simulink model "testemplanner_cs"  (R2020a)
settings: Solver=ode5  StartTime=0.0  StopTime=24  FixedStep=1/1000  RelTol=1e-3
PreLoadFcn:
  | mbxruntime.callbacks.PreLoadFcn(bdroot);
PostLoadFcn:
  | mbxruntime.callbacks.PostLoadFcn(bdroot);
InitFcn:
  | mbxruntime.callbacks.InitFcn(bdroot);
StartFcn:
  | mbxruntime.callbacks.StartFcn(bdroot);
StopFcn:
  | mbxruntime.callbacks.StopFcn(bdroot);
model workspace (MAT data in the model file):
  mbox_table : object (value not decoded)
  model_closed = 0
  sim_status = 0
values from neighbouring files (symbols this model uses):
  c_factor = 43.75    [emplanner_init.m]
  cf = -175016    [emplanner_init.m]
  cr = -130634    [emplanner_init.m]
  global_path_x = [0.057304 1.05668625507 2.05480936558 3.05165624935 4.04722112279 5.04150235808 6.03449985569 7.02621407764 8.01664569183 9.00579544113 9.99366409523 10.9802524329 ... (3001 elements, 3001x1)]    [global_path.mat]
  global_path_y = [8.29 8.29 8.29 8.29 8.29 8.29 8.29 8.29 8.29 8.29 8.29 8.29 ... (3001 elements, 3001x1)]    [global_path.mat]
  KD_PID_distance = 0.0    (= 0)    [emplanner_init.m]
  KD_PID_speed = 0    [emplanner_init.m]
  KI_PID_distance = 0.0    (= 0)    [emplanner_init.m]
  KI_PID_speed = 0    [emplanner_init.m]
  KP_PID_distance = 0.5    [emplanner_init.m]
  KP_PID_speed = 1.8    [emplanner_init.m]
  la = 1.265    [emplanner_init.m]
  lb = 2.947-1.265    (= 1.682)    [emplanner_init.m]
  LQR_K1 = k(:,1)'    [emplanner_init.m]
  LQR_K2 = k(:,2)'    [emplanner_init.m]
  LQR_K3 = k(:,3)'    [emplanner_init.m]
  LQR_K4 = k(:,4)'    [emplanner_init.m]
  m = 2020    [emplanner_init.m]
  rack_displacement = [-39.14 , -37.2 , -35.29 , -33.43 , -31.6 , -29.81 , -28.06 , -26.34 , -24.66 ,      -23.01 , -21.38 , -19.79 , -18.23 , -16.69 , -15.18 , -13.7 , -12.23 , -10.8 , -9.38 , -7.98 ,     -6.61 , -5.25 , -3.91 , -2.59 , -1.29 , 0 , 1.27 , 2.54 , 3.78 , 5.02 , 6.24 , 7.46 , 8.66 ,      9.86 , 11.05 , 12.24 , 13.41 , 14.59 , 15.76 , 16.92 , 18.09 , 19.25 , 20.42 , 21.59 , 22.76 ,      23.93 , 25.11 , 26 ...(+26 chars)    [emplanner_init.m]
  right_wheel_ground = [-70 ,-67.2 , -64.4 , -61.6 , -58.8 , -56 , -53.2 , -50.4 , -47.6 , -44.8 , -42 ,      -39.2 , -36.4 , -33.6 , -30.8 , -28 , -25.2 , -22.4 , -19.6 , -16.8 , -14 , -11.2 , -8.4 , -5.6 ,      -2.8 , 0 , 2.8 , 5.6 , 8.4 , 11.2 , 14 , 16.8 , 19.6 , 22.4 , 25.2 , 28 , 30.8 , 33.6 , 36.4 ,      39.2 , 42 , 44.8 , 47.6 , 50.4 , 53.2 , 56 , 58.8 , 61.6 , 64.4 , 67.2 , 70 ]    [emplanner_init.m]
  vx_break_point = zeros(1,5000)    [emplanner_init.m]
undefined symbols (not defined in the file or in its folder): aubr, DiscIntNeverNeededParam, tablebr, vubr
libraries: PreScanSimulinkLibrary x9, Solver_SF x1, simulink_extras x1
(part 2 of 9)

== system testemplanner_cs/Audi_A8_Sedan_1/control module2 ==
  location_info : Inport
  planning_result : Inport  Port=2
  control_predict_time[s] : Inport  Port=3
  current_time[s] : Inport  Port=4
  Trigger : TriggerPort  TriggerType=function-call  VariantControl=Variant  PortDimensions=1
  Bus Selector1 : BusSelector  OutputSignals=host_x,host_y,host_heading_xy,host_vx,host_vy,host_yawrate,host_speed
  Bus Selector2 : BusSelector  OutputSignals=trajectory_x_gcs,trajectory_y_gcs,trajectory_heading_gcs,trajectory_kappa_gcs,trajectory_speed_gcs,trajectory_accel_gcs,trajectory_time_gcs
  MATLAB Function1 : MATLAB Function  TreatAsAtomicUnit=on
  MATLAB Function2 : MATLAB Function  Commented=on  TreatAsAtomicUnit=on
  control main : Subsystem
  lateral_steer_sw : Outport
  throttle : Outport  Port=2
  brake : Outport  Port=3
  debug_control : Outport  Port=4
  wires:
  [accel] -> control main/13(accelerate_desire[m/s^2])
  [x_r] -> control main/8(xr_desire[m])
  [theta_r] -> control main/10(thetar_desire[rad])
  [y_r] -> control main/9(yr_desire[m])
  [speed] -> control main/12(speed_desire[m/s])
  [kappa_r] -> control main/11(kappar_desire[m^-1])
  MATLAB Function1/4(kappar) -> [kappa_r]
  MATLAB Function1/3(thetar) -> [theta_r]
  MATLAB Function1/2(yr) -> [y_r]
  MATLAB Function1/5(vr) -> [speed]
  MATLAB Function1/6(ar) -> [accel]
  MATLAB Function1/1(xr) -> [x_r]
  current_time[s]/1 -> MATLAB Function1/8(current_time)
  Bus Selector2/1 -> MATLAB Function1/1(trajectory_x)  "<trajectory_x_gcs>"
  Bus Selector2/2 -> MATLAB Function1/2(trajectory_y)  "<trajectory_y_gcs>"
  Bus Selector2/3 -> MATLAB Function1/3(trajectory_heading)  "<trajectory_heading_gcs>"
  Bus Selector2/4 -> MATLAB Function1/4(trajectory_kappa)  "<trajectory_kappa_gcs>"
  Bus Selector2/5 -> MATLAB Function1/5(trajectory_speed)  "<trajectory_speed_gcs>"
  Bus Selector2/6 -> MATLAB Function1/6(trajectory_accel)  "<trajectory_accel_gcs>"
  Bus Selector2/7 -> MATLAB Function1/7(trajectory_time)  "<trajectory_time_gcs>"
  control main/3(brake) -> brake/1
  control main/1(lateral_steer_sw) -> lateral_steer_sw/1
  control main/4(debug_control) -> debug_control/1
  planning_result/1 -> Bus Selector2/1
  control_predict_time[s]/1 -> control main/14(control_predict_time[s])
  location_info/1 -> Bus Selector1/1
  Bus Selector1/3 -> control main/3(host_heading_xy[rad])  "<host_heading_xy>"
  Bus Selector1/6 -> control main/6(host_yawrate[rad/s])  "<host_yawrate>"
  Bus Selector1/1 -> control main/1(host_x[m])  "<host_x>"
  control main/2(throttle) -> throttle/1
  Bus Selector1/7 -> control main/7(host_speed[m/s])  "<host_speed>"
  Bus Selector1/2 -> control main/2(host_y[m])  "<host_y>"
  Bus Selector1/4 -> control main/4(host_vx[m/s])  "<host_vx>"
  Bus Selector1/5 -> control main/5(host_vy[m/s])  "<host_vy>"

== system testemplanner_cs/Audi_A8_Sedan_1/control module3 ==
  location_info : Inport
  planning_result : Inport  Port=2
  control_predict_time[s] : Inport  Port=3
  current_time : Inport  Port=4
  Trigger : TriggerPort  TriggerType=function-call  VariantControl=Variant  PortDimensions=1
  Bus Selector : BusSelector  OutputSignals=trajectory_x_final[m],trajectory_y_final[m],trajectory_heading_final[rad],trajectory_kappa_final[1/m],trajectory_velocity_final[m/s],trajectory_accelerate_final[m/s^2],trajectory_time_final[m/s^2]
  Bus Selector1 : BusSelector  OutputSignals=host_x,host_y,host_heading_xy,host_vx,host_vy,host_yawrate,host_speed
  MATLAB Function : MATLAB Function  TreatAsAtomicUnit=on
  control main : Subsystem
  lateral_steer_sw : Outport
  throttle : Outport  Port=2
  brake : Outport  Port=3
  debug_control : Outport  Port=4
  wires:
  [trajecotory_x] -> MATLAB Function/1(trajectory_x)
  [trajecotory_y] -> MATLAB Function/2(trajectory_y)
  [trajecotory_heading] -> MATLAB Function/3(trajectory_heading)
  [trajecotory_kappa] -> MATLAB Function/4(trajectory_kappa)
  [trajecotory_speed] -> MATLAB Function/5(trajectory_speed)
  [trajecotory_accel] -> MATLAB Function/6(trajectory_accel)
  [trajecotory_time] -> MATLAB Function/7(trajectory_time)
  Bus Selector/7 -> [trajecotory_time]  "<trajectory_time_final[m/s^2]>"
  Bus Selector/6 -> [trajecotory_accel]  "<trajectory_accelerate_final[m/s^2]>"
  Bus Selector/5 -> [trajecotory_speed]  "<trajectory_velocity_final[m/s]>"
  Bus Selector/4 -> [trajecotory_kappa]  "<trajectory_kappa_final[1/m]>"
  Bus Selector/3 -> [trajecotory_heading]  "<trajectory_heading_final[rad]>"
  Bus Selector/2 -> [trajecotory_y]  "<trajectory_y_final[m]>"
  Bus Selector/1 -> [trajecotory_x]  "<trajectory_x_final[m]>"
  planning_result/1 -> Bus Selector/1
  current_time/1 -> MATLAB Function/8(current_time)
  MATLAB Function/1(xr) -> control main/8(xr_desire[m])
  MATLAB Function/2(yr) -> control main/9(yr_desire[m])
  MATLAB Function/3(thetar) -> control main/10(thetar_desire[rad])
  MATLAB Function/4(kappar) -> control main/11(kappar_desire[m^-1])
  MATLAB Function/5(vr) -> control main/12(speed_desire[m/s])
  MATLAB Function/6(ar) -> control main/13(accelerate_desire[m/s^2])
  control main/3(brake) -> brake/1
  control main/1(lateral_steer_sw) -> lateral_steer_sw/1
  control main/4(debug_control) -> debug_control/1
  control_predict_time[s]/1 -> control main/14(control_predict_time[s])
  location_info/1 -> Bus Selector1/1
  Bus Selector1/3 -> control main/3(host_heading_xy[rad])  "<host_heading_xy>"
  Bus Selector1/6 -> control main/6(host_yawrate[rad/s])  "<host_yawrate>"
  Bus Selector1/1 -> control main/1(host_x[m])  "<host_x>"
  control main/2(throttle) -> throttle/1
  Bus Selector1/7 -> control main/7(host_speed[m/s])  "<host_speed>"
  Bus Selector1/2 -> control main/2(host_y[m])  "<host_y>"
  Bus Selector1/4 -> control main/4(host_vx[m/s])  "<host_vx>"
  Bus Selector1/5 -> control main/5(host_vy[m/s])  "<host_vy>"

== system testemplanner_cs/Audi_A8_Sedan_1/decision&planning module ==
  note: 灰色的函数为通用算法函数，可以在多个模块复用
  location_info : Inport
  routine_info : Inport  Port=2
  perceptiong_result : Inport  Port=3
  current_time : Inport  Port=4
  pre_planning_result : Inport  Port=5
  Trigger : TriggerPort  TriggerType=function-call  VariantControl=Variant  PortDimensions=1
  Bus Creator : BusCreator  Inputs=1
  Bus Creator1 : BusCreator  Inputs=4
  EM Planner : Subsystem
  EM_planner1 : Subsystem  Commented=on
  referenceline provider : Subsystem
  planning_result : Outport
  debug_planning : Outport  Port=2
  wires:
  [planning_info] -> planning_result/1
  referenceline provider/2(referenceline_y[m]) -> [referenceline_y]
  routine_info/1 -> [routine_info]
  [routine_info] -> referenceline provider/2(routine_info)
  referenceline provider/5(referenceline_debug) -> [referenceline_debug]
  referenceline provider/4(referenceline_kappa[rad/m]) -> [referenceline_kappa]
  referenceline provider/1(referenceline_x[m]) -> [referenceline_x]
  [Location_info] -> referenceline provider/1(location_info)
  location_info/1 -> [Location_info]
  referenceline provider/3(referenceline_heading[rad]) -> [referenceline_heading]
  [referenceline_debug] -> Bus Creator/1  "debug_referenceline"
  Bus Creator/1 -> debug_planning/1
  perceptiong_result/1 -> [perceptiong_result]
  [referenceline_kappa] -> Bus Creator1/4
  [referenceline_x] -> Bus Creator1/1
  [referenceline_heading] -> Bus Creator1/3
  [referenceline_y] -> Bus Creator1/2
  Bus Creator1/1 -> [referenceline_info]
  [Location_info] -> EM Planner/2(location info)
  [referenceline_info] -> EM Planner/1(referenceline info)
  [perceptiong_result] -> EM Planner/3(perception info)
  current_time/1 -> [current_time]
  pre_planning_result/1 -> [pre_planning_result]
  [current_time] -> EM Planner/5(current time)
  [pre_planning_result] -> EM Planner/4(pre_planning info)
  EM Planner/1(EM Planner result) -> [planning_info]

== system testemplanner_cs/Audi_A8_Sedan_1/location module ==
  host_x[m] : Inport
  host_y[m] : Inport  Port=2
  host_heading_xy[rad] : Inport  Port=3
  host_vx[m/s] : Inport  Port=4
  host_vy[m/s] : Inport  Port=5
  host_yawrate[rad/s] : Inport  Port=6
  host_speed[m/s] : Inport  Port=7
  host_ax[m·s(-2)] : Inport  Port=8
  host_ay[m·s(-2)] : Inport  Port=9
  Bus Creator : BusCreator  Inputs=9
  location_Info : Outport
  wires:
  host_yawrate[rad/s]/1 -> Bus Creator/6  "host_yawrate"
  host_vy[m/s]/1 -> Bus Creator/5  "host_vy"
  host_heading_xy[rad]/1 -> Bus Creator/3  "host_heading_xy"
  host_speed[m/s]/1 -> Bus Creator/7  "host_speed"
  Bus Creator/1 -> location_Info/1
  host_y[m]/1 -> Bus Creator/2  "host_y"
  host_x[m]/1 -> Bus Creator/1  "host_x"
  host_vx[m/s]/1 -> Bus Creator/4  "host_vx"
  host_ay[m·s(-2)]/1 -> Bus Creator/9  "host_ay"
  host_ax[m·s(-2)]/1 -> Bus Creator/8  "host_ax"

== system testemplanner_cs/Audi_A8_Sedan_1/routine module ==
  Bus Creator : BusCreator  Inputs=2
  Constant : Constant  Value=global_path_x
  Constant1 : Constant  Value=global_path_y
  global_path_info : Outport
  wires:
  Constant/1 -> [global_path_x]
  Constant1/1 -> [global_path_y]
  [global_path_x] -> Bus Creator/1  "global_path_x"
  [global_path_y] -> Bus Creator/2  "global_path_y"
  Bus Creator/1 -> global_path_info/1

== system testemplanner_cs/Box_1/Dynamics_Empty ==
  note: For state mode 'Dynamic' positions
      | are not taken into account, as they
      | are computed by integrating velocity.
      | Click annotation for Help.
  Ground_{1..9} (9 alike) : Ground
  MuxState : Subsystem  Tag=mux/State  mask(Empty Dynamics State Block){positioningmode=on, TimeStep=50/1000}
      mask prompts: positioningmode "Positioning Mode"; TimeStep "Auto Assigned: Time Step [s]"
      mask help:
      | Build the state of an actor based on user input.
      | The user can either use positioning mode or dynamics mode.
      | - When using positioning mode the position and orientation of the actor are set directly based on the input. Expected input is relative to the initial position and orientation of the actor. It's also possible to specify the velocity of the actor, though this input isn't used, only passed on.
      | - When using dynamics mode the position input is ignored. Expected input is velocity and orientation. The velocity is relative the current orientation of the actor, while orientation is relative to its initial orientation. The position of the actor is calculated based on the velocity and orientation given.
      settings: DeleteFcn=PreScanBlockDeleteFcn;
  State : Outport  Tag=outport/StateOutport  SampleTime=50/1000
  wires:
  MuxState/1(state) -> State/1
  Ground_1/1 -> MuxState/1(x [m])
  Ground_2/1 -> MuxState/2(y [m])
  Ground_3/1 -> MuxState/3(z [m])
  Ground_4/1 -> MuxState/4(dx [m/s])
  Ground_5/1 -> MuxState/5(dy [m/s])
  Ground_6/1 -> MuxState/6(dz [m/s])
  Ground_7/1 -> MuxState/7(R [rad])
  Ground_8/1 -> MuxState/8(P [rad])
  Ground_9/1 -> MuxState/9(Y [rad])

== system testemplanner_cs/Box_1/SELF_Demux ==
  SELF : Inport  OutDataTypeStr=Bus: PRESCAN_SELFSENSORDATA
  Bus Selector : BusSelector  OutputSignals=PositionX,PositionY,PositionZ,OrientationRoll,OrientationPitch,OrientationYaw,Velocity,Yaw_rate,Lat,Long,Alt
  Demux2 : Demux  Outputs=3
  Gain : Gain  Gain=180/pi
  Gain1 : Gain  Gain=180/pi
  Vector Concatenate1 : Concatenate  NumInputs=3
  compas converter : Subsystem
  x [m] : Outport
  y [m] : Outport  Port=2
  z [m] : Outport  Port=3
  rotx [deg] : Outport  Port=4
  roty [deg] : Outport  Port=5
  rotz [deg] : Outport  Port=6
  GPS lat [deg] : Outport  Port=7
  GPS long [deg] : Outport  Port=8
  GPS alt [m] : Outport  Port=9
  velocity [m/s] : Outport  Port=10
  heading [deg] : Outport  Port=11
  yaw rate [deg/s] : Outport  Port=12
  wires:
  Bus Selector/11 -> GPS alt [m]/1  "<Alt>"
  Bus Selector/10 -> GPS long [deg]/1  "<Long>"
  Bus Selector/9 -> GPS lat [deg]/1  "<Lat>"
  Bus Selector/8 -> Gain1/1  "<Yaw_rate>"
  Bus Selector/7 -> velocity [m/s]/1  "<Velocity>"
  Bus Selector/6 -> compas converter/1(rotz [rad]), Vector Concatenate1/3  "<OrientationYaw>"
  Bus Selector/5 -> Vector Concatenate1/2  "<OrientationPitch>"
  Bus Selector/4 -> Vector Concatenate1/1  "<OrientationRoll>"
  Vector Concatenate1/1 -> Gain/1
  Bus Selector/3 -> z [m]/1  "<PositionZ>"
  Bus Selector/2 -> y [m]/1  "<PositionY>"
  Bus Selector/1 -> x [m]/1  "<PositionX>"
  SELF/1 -> Bus Selector/1
  Gain/1 -> Demux2/1
  Demux2/1 -> rotx [deg]/1
  Demux2/2 -> roty [deg]/1
  Demux2/3 -> rotz [deg]/1
  compas converter/1(heading [deg]) -> heading [deg]/1
  Gain1/1 -> yaw rate [deg/s]/1

== system testemplanner_cs/Box_1/STATE_Box_1 ==
  State : Inport  SampleTime=TimeStep
  Bus Creator : BusCreator  Inputs=15  OutDataTypeStr=Bus: PRESCAN_STATEACTUATORDATA  NonVirtualBus=on
  Demux : Demux  Outputs=15
  iniBODYAngles wrtVEH [rad] : Constant  Value=[Roll0 Pitch0 0]  SampleTime=TimeStep
  iniVEHAngles wrtGLOB [rad] : Constant  Value=[0 0 Yaw0]  SampleTime=TimeStep
  iniVEHposition wrtGLOB [m] : Constant  Value=[x0 y0 z0]  SampleTime=TimeStep
  state2FullState : PreScanSimulinkLibrary/state2FullState  SystemSampleTime=-1  Latency=0  AutoFrameSizeCalculation=off
  StateBus : Outport  OutDataTypeStr=Bus: PRESCAN_STATEACTUATORDATA
  wires:
  Bus Creator/1 -> StateBus/1
  State/1 -> state2FullState/1
  state2FullState/1 -> Demux/1
  iniVEHposition wrtGLOB [m]/1 -> state2FullState/2
  iniBODYAngles wrtVEH [rad]/1 -> state2FullState/3
  iniVEHAngles wrtGLOB [rad]/1 -> state2FullState/4
  Demux/1 -> Bus Creator/1  "PositionX"
  Demux/2 -> Bus Creator/2  "PositionY"
  Demux/3 -> Bus Creator/3  "PositionZ"
  Demux/4 -> Bus Creator/4  "VelocityX"
  Demux/5 -> Bus Creator/5  "VelocityY"
  Demux/6 -> Bus Creator/6  "VelocityZ"
  Demux/7 -> Bus Creator/7  "AccelerationX"
  Demux/8 -> Bus Creator/8  "AccelerationY"
  Demux/9 -> Bus Creator/9  "AccelerationZ"
  Demux/10 -> Bus Creator/10  "OrientationRoll"
  Demux/11 -> Bus Creator/11  "OrientationPitch"
  Demux/12 -> Bus Creator/12  "OrientationYaw"
  Demux/13 -> Bus Creator/13  "AngularVelocityRoll"
  Demux/14 -> Bus Creator/14  "AngularVelocityPitch"
  Demux/15 -> Bus Creator/15  "AngularVelocityYaw"

== system testemplanner_cs/Audi_A8_Sedan_1/AIR_1_Demux/Activate_Switch ==
  BeamID : Inport
  Heading : Inport  Port=2
  Constant : Constant  Value=0
  Product1 : Product  RndMeth=Zero
  Relational Operator : RelationalOperator  Operator=~=  OutDataTypeStr=boolean  RndMeth=Nearest
  On/Off : Outport
  wires:
  Constant/1 -> Relational Operator/1
  Relational Operator/1 -> Product1/1
  BeamID/1 -> Relational Operator/2
  Product1/1 -> On/Off/1
  Heading/1 -> Product1/2

== system testemplanner_cs/Audi_A8_Sedan_1/AIR_1_Demux/Signal2ArrayOfSignals1 ==
  note: Set mask parameter VECTORLENGTH
      |  to MAXMESSAGES
  note: Initial state of Previous vector block
      | set to zeros(VECTORLENGTH,1)
  LoopIndex : Inport
  Element : Inport  Port=2
  Assignment : Assignment  IndexOptions=Index vector (port)  Indices=1  OutputSizes=1
  Previous vector : Memory  InitialCondition=zeros(VECTORLENGTH,1)  InheritSampleTime=on
  ArrayofElements : Outport
  wires:
  Element/1 -> Assignment/2
  LoopIndex/1 -> Assignment/3
  Previous vector/1 -> Assignment/1
  Assignment/1 -> ArrayofElements/1, Previous vector/1

== system testemplanner_cs/Audi_A8_Sedan_1/AIR_1_Demux/Signal2ArrayOfSignals2 ==
  note: Set mask parameter VECTORLENGTH
      |  to MAXMESSAGES
  note: Initial state of Previous vector block
      | set to zeros(VECTORLENGTH,1)
  LoopIndex : Inport
  Element : Inport  Port=2
  Assignment : Assignment  IndexOptions=Index vector (port)  Indices=1  OutputSizes=1
  Previous vector : Memory  InitialCondition=zeros(VECTORLENGTH,1)  InheritSampleTime=on
  ArrayofElements : Outport
  wires:
  Element/1 -> Assignment/2
  LoopIndex/1 -> Assignment/3
  Previous vector/1 -> Assignment/1
  Assignment/1 -> ArrayofElements/1, Previous vector/1

== system testemplanner_cs/Audi_A8_Sedan_1/AIR_1_Demux/Signal2ArrayOfSignals3 ==
  note: Set mask parameter VECTORLENGTH
      |  to MAXMESSAGES
  note: Initial state of Previous vector block
      | set to zeros(VECTORLENGTH,1)
  LoopIndex : Inport
  Element : Inport  Port=2
  Assignment : Assignment  IndexOptions=Index vector (port)  Indices=1  OutputSizes=1
  Previous vector : Memory  InitialCondition=zeros(VECTORLENGTH,1)  InheritSampleTime=on
  ArrayofElements : Outport
  wires:
  Element/1 -> Assignment/2
  LoopIndex/1 -> Assignment/3
  Previous vector/1 -> Assignment/1
  Assignment/1 -> ArrayofElements/1, Previous vector/1

== system testemplanner_cs/Audi_A8_Sedan_1/AIR_1_Demux/Signal2ArrayOfSignals4 ==
  note: Set mask parameter VECTORLENGTH
      |  to MAXMESSAGES
  note: Initial state of Previous vector block
      | set to zeros(VECTORLENGTH,1)
  LoopIndex : Inport
  Element : Inport  Port=2
  Assignment : Assignment  IndexOptions=Index vector (port)  Indices=1  OutputSizes=1
  Previous vector : Memory  InitialCondition=zeros(VECTORLENGTH,1)  InheritSampleTime=on
  ArrayofElements : Outport
  wires:
  Element/1 -> Assignment/2
  LoopIndex/1 -> Assignment/3
  Previous vector/1 -> Assignment/1
  Assignment/1 -> ArrayofElements/1, Previous vector/1

== system testemplanner_cs/Audi_A8_Sedan_1/AIR_1_Demux/Signal2ArrayOfSignals5 ==
  note: Set mask parameter VECTORLENGTH
      |  to MAXMESSAGES
  note: Initial state of Previous vector block
      | set to zeros(VECTORLENGTH,1)
  LoopIndex : Inport
  Element : Inport  Port=2
  Assignment : Assignment  IndexOptions=Index vector (port)  Indices=1  OutputSizes=1
  Previous vector : Memory  InitialCondition=zeros(VECTORLENGTH,1)  InheritSampleTime=on
  ArrayofElements : Outport
  wires:
  Element/1 -> Assignment/2
  LoopIndex/1 -> Assignment/3
  Previous vector/1 -> Assignment/1
  Assignment/1 -> ArrayofElements/1, Previous vector/1

== system testemplanner_cs/Audi_A8_Sedan_1/AIR_1_Demux/Signal2ArrayOfSignals6 ==
  note: Set mask parameter VECTORLENGTH
      |  to MAXMESSAGES
  note: Initial state of Previous vector block
      | set to zeros(VECTORLENGTH,1)
  LoopIndex : Inport
  Element : Inport  Port=2
  Assignment : Assignment  IndexOptions=Index vector (port)  Indices=1  OutputSizes=1
  Previous vector : Memory  InitialCondition=zeros(VECTORLENGTH,1)  InheritSampleTime=on
  ArrayofElements : Outport
  wires:
  Element/1 -> Assignment/2
  LoopIndex/1 -> Assignment/3
  Previous vector/1 -> Assignment/1
  Assignment/1 -> ArrayofElements/1, Previous vector/1

== system testemplanner_cs/Audi_A8_Sedan_1/Dynamics_UserSpecified/CarSim2PreScanSTATE ==
  CarSim_In : Inport
  D2R : Gain  Gain=pi/180
  Demux : Demux  Outputs=[3 3 3 -1]
  Demux1 : Demux  Outputs=3
  Demux2 : Demux  Outputs=3
  Demux3 : Demux  Outputs=3
  Demux4 : Demux  Outputs=28
  Gain : Gain  Gain=9.8
  Gain1 : Gain  Gain=9.8
  Terminator_{1..26} (26 alike) : Terminator
  Transformation_SprungMassCarSim2PreScan : Subsystem
  km|h_to_m|s : Gain  Gain=1/3.6
  x [m] : Outport
  y [m] : Outport  Port=2
  z [m] : Outport  Port=3
  dx [m/s] : Outport  Port=4
  dy [m/s] : Outport  Port=5
  dz [m/s] : Outport  Port=6
  R [rad] : Outport  Port=7
  P [rad] : Outport  Port=8
  Y [rad] : Outport  Port=9
  ax [m/s^2] : Outport  Port=10
  ay [m/s^2] : Outport  Port=11
  wires:
  Demux/4 -> Demux4/1
  Demux3/3 -> Y [rad]/1
  Demux3/2 -> P [rad]/1
  Demux3/1 -> R [rad]/1
  Demux2/3 -> dz [m/s]/1
  Demux2/2 -> dy [m/s]/1
  Demux2/1 -> dx [m/s]/1
  Demux1/3 -> z [m]/1
  Demux1/2 -> y [m]/1
  Demux1/1 -> x [m]/1
  Transformation_SprungMassCarSim2PreScan/1(Out1) -> Demux1/1
  Demux/1 -> Transformation_SprungMassCarSim2PreScan/1(In1)
  CarSim_In/1 -> Demux/1
  km|h_to_m|s/1 -> Demux2/1
  Demux/2 -> km|h_to_m|s/1
  Demux/3 -> D2R/1
  D2R/1 -> Demux3/1
  Demux4/28 -> Gain1/1
  Demux4/27 -> Gain/1
  Gain/1 -> ax [m/s^2]/1
  Gain1/1 -> ay [m/s^2]/1
  Demux4/1 -> Terminator_1/1
  Demux4/2 -> Terminator_2/1
  Demux4/3 -> Terminator_3/1
  Demux4/4 -> Terminator_4/1
  Demux4/5 -> Terminator_5/1
  Demux4/6 -> Terminator_6/1
  Demux4/7 -> Terminator_7/1
  Demux4/8 -> Terminator_8/1
  Demux4/9 -> Terminator_9/1
  Demux4/10 -> Terminator_10/1
  Demux4/11 -> Terminator_11/1
  Demux4/12 -> Terminator_12/1
  Demux4/13 -> Terminator_13/1
  Demux4/14 -> Terminator_14/1
  Demux4/15 -> Terminator_15/1
  Demux4/16 -> Terminator_16/1
  Demux4/17 -> Terminator_17/1
  Demux4/18 -> Terminator_18/1
  Demux4/19 -> Terminator_19/1
  Demux4/20 -> Terminator_20/1
  Demux4/21 -> Terminator_21/1
  Demux4/22 -> Terminator_22/1
  Demux4/23 -> Terminator_23/1
  Demux4/24 -> Terminator_24/1
  Demux4/25 -> Terminator_25/1
  Demux4/26 -> Terminator_26/1

== system testemplanner_cs/Audi_A8_Sedan_1/Dynamics_UserSpecified/MuxState ==
  note: mode: Dynamics
  note: mode: Positioning
  note: mode: Dynamics
      | VelVEHICLE
      | wrt VEH
  note: AnglesVEHICLE
      | wrtGLOB
  note: For state mode 'Dynamic' positions
      | are not taken into account, as they
      | are computed by integrating velocity.
      | Click annotation for Help.
  x [m] : Inport  SampleTime=TimeStep
  y [m] : Inport  Port=2  SampleTime=TimeStep
  z [m] : Inport  Port=3  SampleTime=TimeStep
  dx [m/s] : Inport  Port=4  SampleTime=TimeStep
  dy [m/s] : Inport  Port=5  SampleTime=TimeStep
  dz [m/s] : Inport  Port=6  SampleTime=TimeStep
  R [rad] : Inport  Port=7  SampleTime=TimeStep
  P [rad] : Inport  Port=8  SampleTime=TimeStep
  Y [rad] : Inport  Port=9  SampleTime=TimeStep
  Constant : Constant  DisableCoverage=on  Value=positioningmode
  Discrete-Time Integrator : DiscreteIntegrator  SampleTime=TimeStep  ICPrevOutput=DiscIntNeverNeededParam  ICPrevScaledInput=DiscIntNeverNeededParam
  Ground : Ground
  Ground1 : Ground
  Mux1 : Mux  Inputs=[3 3]
  Mux2 : Mux  Inputs=3
  Mux3 : Mux  Inputs=3
  Mux4 : Mux  Inputs=3
  Mux5 : Mux  Inputs=[3 3]
  Mux6 : Mux  Inputs=[6 3]
  Switch : Switch  Threshold=0.5
  Transformation_BODY2GLOBAL : PreScanSimulinkLibrary/Simple_Vehicle_Dynamics/Chassis/MuxDynState/Transformation_BODY2GLOBAL  SystemSampleTime=-1  Latency=0  AutoFrameSizeCalculation=off
  mux3 : Mux  Inputs=3
  state : Outport
  wires:
  Constant/1 -> Switch/2
  Mux6/1 -> state/1
  Mux4/1 -> Mux1/1
  Mux5/1 -> Switch/3
  Mux1/1 -> Switch/1
  Switch/1 -> Mux6/1  "PosVeh wrt  GLOB"
  P [rad]/1 -> Mux3/2
  R [rad]/1 -> Mux3/1
  dz [m/s]/1 -> Mux2/3
  dy [m/s]/1 -> Mux2/2
  dx [m/s]/1 -> Mux2/1
  z [m]/1 -> Mux4/3
  y [m]/1 -> Mux4/2
  x [m]/1 -> Mux4/1
  Ground1/1 -> mux3/2  "pitch"
  Y [rad]/1 -> mux3/3, Mux3/3  "yaw"
  Mux3/1 -> Mux6/2
  Transformation_BODY2GLOBAL/1 -> Discrete-Time Integrator/1, Mux5/2  "VelVEH wrt  GLOB"
  mux3/1 -> Transformation_BODY2GLOBAL/2
  Ground/1 -> mux3/1  "roll"
  Mux2/1 -> Mux1/2, Transformation_BODY2GLOBAL/1
  Discrete-Time Integrator/1 -> Mux5/1  "PosVEH wrt  GLOB"

== system testemplanner_cs/Audi_A8_Sedan_1/SELF_Demux/compas converter ==
  rotz [rad] : Inport
  cart2compas : Subsystem
  rad2deg : Gain  Gain=180/pi
  heading [deg] : Outport
  wires:
  rad2deg/1 -> cart2compas/1(Angle [deg])
  rotz [rad]/1 -> rad2deg/1
  cart2compas/1(heading [deg]) -> heading [deg]/1

== system testemplanner_cs/Audi_A8_Sedan_1/Trajectories/Traj2State1 ==
  Traj Org : Inport
  Offset : Inport  Port=2
  Add2 : Sum
  ApplyRotation : PreScanSimulinkLibrary/ApplyRotation  SystemSampleTime=-1  Latency=0  AutoFrameSizeCalculation=off
  ApplyRotation1 : PreScanSimulinkLibrary/ApplyRotation  SystemSampleTime=-1  Latency=0  AutoFrameSizeCalculation=off
  ApplyRotation2 : PreScanSimulinkLibrary/ApplyRotation  SystemSampleTime=-1  Latency=0  AutoFrameSizeCalculation=off
  Constant : Constant  Value=zeros(12,1)
  Mux : Mux  Inputs=6
  Mux1 : Mux  Inputs=2
  Mux{2,4..9} (7 alike) : Mux  Inputs=3
  Mux3 : Mux  Inputs=2
  Selector : Selector  InputPortWidth=6  IndexOptions=Index vector (dialog)  Indices=[4 5 6]  OutputSizes=1
  Selector1 : Selector  InputPortWidth=21  IndexOptions=Index vector (dialog)  Indices=[5]  OutputSizes=1
  Selector10 : Selector  InputPortWidth=21  IndexOptions=Index vector (dialog)  Indices=[2]  OutputSizes=1
  Selector11 : Selector  InputPortWidth=21  IndexOptions=Index vector (dialog)  Indices=[3]  OutputSizes=1
  Selector12 : Selector  InputPortWidth=21  IndexOptions=Index vector (dialog)  Indices=[1]  OutputSizes=1
  Selector13 : Selector  InputPortWidth=21  IndexOptions=Index vector (dialog)  Indices=[8]  OutputSizes=1
  Selector14 : Selector  InputPortWidth=21  IndexOptions=Index vector (dialog)  Indices=[9]  OutputSizes=1
  Selector15 : Selector  InputPortWidth=21  IndexOptions=Index vector (dialog)  Indices=[7]  OutputSizes=1
  Selector16 : Selector  InputPortWidth=21  IndexOptions=Index vector (dialog)  Indices=[14]  OutputSizes=1
  Selector17 : Selector  InputPortWidth=21  IndexOptions=Index vector (dialog)  Indices=[15]  OutputSizes=1
  Selector18 : Selector  InputPortWidth=21  IndexOptions=Index vector (dialog)  Indices=[13]  OutputSizes=1
  Selector19 : Selector  InputPortWidth=21  IndexOptions=Index vector (dialog)  Indices=[20]  OutputSizes=1
  Selector2 : Selector  InputPortWidth=21  IndexOptions=Index vector (dialog)  Indices=[6]  OutputSizes=1
  Selector20 : Selector  InputPortWidth=21  IndexOptions=Index vector (dialog)  Indices=[21]  OutputSizes=1
  Selector21 : Selector  InputPortWidth=21  IndexOptions=Index vector (dialog)  Indices=[19]  OutputSizes=1
  Selector3 : Selector  InputPortWidth=21  IndexOptions=Index vector (dialog)  Indices=[12]  OutputSizes=1
  Selector4 : Selector  InputPortWidth=21  IndexOptions=Index vector (dialog)  Indices=[17]  OutputSizes=1
  Selector5 : Selector  InputPortWidth=21  IndexOptions=Index vector (dialog)  Indices=[18]  OutputSizes=1
  Selector6 : Selector  InputPortWidth=21  IndexOptions=Index vector (dialog)  Indices=[16]  OutputSizes=1
  Selector7 : Selector  InputPortWidth=21  IndexOptions=Index vector (dialog)  Indices=[11]  OutputSizes=1
  Selector8 : Selector  InputPortWidth=21  IndexOptions=Index vector (dialog)  Indices=[10]  OutputSizes=1
  Selector9 : Selector  InputPortWidth=21  IndexOptions=Index vector (dialog)  Indices=[4]  OutputSizes=1
  Traj2State2 : Subsystem
  state : Outport
  wires:
  Mux9/1 -> ApplyRotation2/2, ApplyRotation1/2, ApplyRotation/2
  Selector20/1 -> Mux9/3
  Selector19/1 -> Mux9/2
  Selector21/1 -> Mux9/1
  Selector5/1 -> Mux8/3
  Selector4/1 -> Mux8/2
  Selector6/1 -> Mux8/1
  Mux8/1 -> Mux/6
  Mux6/1 -> ApplyRotation2/1
  Mux7/1 -> Mux/4
  ApplyRotation2/1 -> Mux/5
  Selector3/1 -> Mux7/3
  Selector7/1 -> Mux7/2
  Selector8/1 -> Mux7/1
  Mux4/1 -> Mux/2
  Mux5/1 -> ApplyRotation1/1
  ApplyRotation1/1 -> Mux/3
  Mux2/1 -> ApplyRotation/1
  ApplyRotation/1 -> Mux/1
  Selector2/1 -> Mux4/3
  Selector1/1 -> Mux4/2
  Selector9/1 -> Mux4/1
  Selector17/1 -> Mux6/3
  Selector16/1 -> Mux6/2
  Selector18/1 -> Mux6/1
  Selector14/1 -> Mux5/3
  Selector13/1 -> Mux5/2
  Selector15/1 -> Mux5/1
  Selector11/1 -> Mux2/3
  Selector10/1 -> Mux2/2
  Selector12/1 -> Mux2/1
  Mux3/1 -> Selector8/1, Selector7/1, Selector3/1, Selector18/1, Selector16/1, Selector17/1, Selector6/1, Selector20/1, Selector19/1, Selector21/1, Selector5/1, Selector4/1, Selector14/1, Selector13/1, Selector15/1, Selector2/1, Selector1/1, Selector9/1, Selector12/1, Selector10/1, Selector11/1
  Mux1/1 -> Add2/2
  Constant/1 -> Mux1/2
  Add2/1 -> Traj2State2/1(traj)
  Selector/1 -> Mux3/2
  Traj Org/1 -> Mux3/1
  Offset/1 -> Mux1/1, Selector/1
  Mux/1 -> Add2/1
  Traj2State2/1(state) -> state/1

== system testemplanner_cs/Audi_A8_Sedan_1/Trajectories/TrajCoGOffset ==
  State In : Inport
  Add : Sum  Inputs=+-+
  Add1 : Sum
  ApplyRotation : PreScanSimulinkLibrary/ApplyRotation  SystemSampleTime=-1  Latency=0  AutoFrameSizeCalculation=off
  ApplyRotation1 : PreScanSimulinkLibrary/ApplyRotation  SystemSampleTime=-1  Latency=0  AutoFrameSizeCalculation=off
  CoG Offset : Constant  Value=[0 0 CoGOffsetZ]
  Degrees to Radians : simulink_extras/Transformations/Degrees to Radians
  Demux1 : Demux  Outputs=[3 3 3]
  Mux : Mux  Inputs=[3 3 3]
  Orientation : Constant  Value=[InitRoll InitPitch 0]
  State Out : Outport
  wires:
  State In/1 -> Demux1/1
  Demux1/1 -> Add/1
  Add/1 -> Mux/1
  Demux1/3 -> Mux/3, Add1/2
  Mux/1 -> State Out/1
  Demux1/2 -> Mux/2
  Orientation/1 -> Degrees to Radians/1
  ApplyRotation/1 -> Add/3
  ApplyRotation1/1 -> Add/2
  Add1/1 -> ApplyRotation/2
  CoG Offset/1 -> ApplyRotation1/1, ApplyRotation/1
  Degrees to Radians/1 -> Add1/1, ApplyRotation1/2

== system testemplanner_cs/Audi_A8_Sedan_1/Trajectories/Trajectory_1 ==
  From Workspace : FromWorkspace  VariableName=trajectory  SampleTime=TimeStep  ZeroCross=off  OutputAfterFinalValue=Holding final value
  From Workspace1 : FromWorkspace  VariableName=trajectory  SampleTime=TimeStep  ZeroCross=off  OutputAfterFinalValue=Setting to zero
  Mux : Mux  Inputs=2
  Selector1 : Selector  InputPortWidth=24  IndexOptions=Index vector (dialog)  Indices=[7:18]  OutputSizes=1
  Selector9 : Selector  InputPortWidth=24  IndexOptions=Index vector (dialog)  Indices=[1:6]  OutputSizes=1
  trajectory : Outport
  wires:
  From Workspace/1 -> Selector9/1
  From Workspace1/1 -> Selector1/1
  Mux/1 -> trajectory/1
  Selector9/1 -> Mux/1
  Selector1/1 -> Mux/2

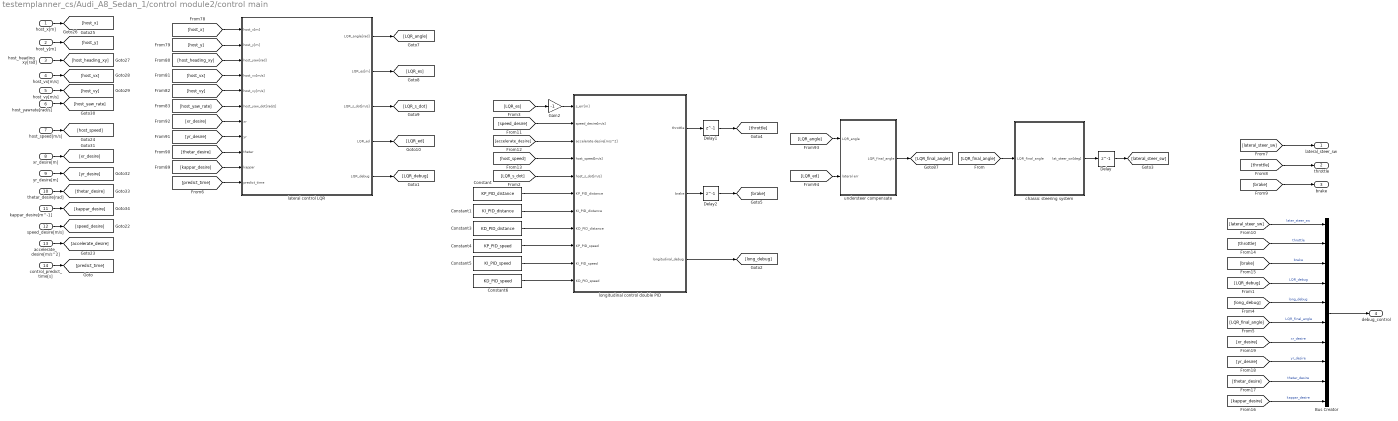
== system testemplanner_cs/Audi_A8_Sedan_1/control module2/control main ==
  host_x[m] : Inport
  host_y[m] : Inport  Port=2
  host_heading_xy[rad] : Inport  Port=3
  host_vx[m/s] : Inport  Port=4
  host_vy[m/s] : Inport  Port=5
  host_yawrate[rad/s] : Inport  Port=6
  host_speed[m/s] : Inport  Port=7
  xr_desire[m] : Inport  Port=8
  yr_desire[m] : Inport  Port=9
  thetar_desire[rad] : Inport  Port=10
  kappar_desire[m^-1] : Inport  Port=11
  speed_desire[m/s] : Inport  Port=12
  accelerate_desire[m/s^2] : Inport  Port=13
  control_predict_time[s] : Inport  Port=14
  Bus Creator : BusCreator  Inputs=10
  Constant : Constant  Value=KP_PID_distance
  Constant1 : Constant  Value=KI_PID_distance
  Constant3 : Constant  Value=KD_PID_distance
  Constant4 : Constant  Value=KP_PID_speed
  Constant5 : Constant  Value=KI_PID_speed
  Constant6 : Constant  Value=KD_PID_speed
  Delay : Delay  DelayLength=1
  Delay1 : Delay  DelayLength=1
  Delay2 : Delay  DelayLength=1
  Gain2 : Gain  Gain=-1
  chassic steering system : Subsystem
  lateral control LQR : Subsystem
  longitudinal control double PID : Subsystem
  understeer compensate : Subsystem
  lateral_steer_sw : Outport
  throttle : Outport  Port=2
  brake : Outport  Port=3
  debug_control : Outport  Port=4
  wires:
  [kappar_desire] -> Bus Creator/10  "kappar_desire"
  [thetar_desire] -> Bus Creator/9  "thetar_desire"
  [yr_desire] -> Bus Creator/8  "yr_desire"
  [xr_desire] -> Bus Creator/7  "xr_desire"
  Bus Creator/1 -> debug_control/1
  [LQR_final_angle] -> Bus Creator/6  "LQR_final_angle"
  [long_debug] -> Bus Creator/5  "long_debug"
  [LQR_debug] -> Bus Creator/4  "LQR_debug"
  [brake] -> Bus Creator/3  "brake"
  [throttle] -> Bus Creator/2  "throttle"
  [lateral_steer_sw] -> Bus Creator/1  "later_steer_sw"
  [brake] -> brake/1
  [throttle] -> throttle/1
  [lateral_steer_sw] -> lateral_steer_sw/1
  Delay2/1 -> [brake]
  Delay1/1 -> [throttle]
  Delay/1 -> [lateral_steer_sw]
  longitudinal control double PID/3(longitudinal_debug) -> [long_debug]
  lateral control LQR/5(LQR_debug) -> [LQR_debug]
  longitudinal control double PID/2(brake) -> Delay2/1
  longitudinal control double PID/1(throttle) -> Delay1/1
  chassic steering system/1(lat_steer_sw[deg]) -> Delay/1
  [LQR_final_angle] -> chassic steering system/1(LQR_final_angle)
  [LQR_es] -> Gain2/1
  Gain2/1 -> longitudinal control double PID/1(s_err[m])
  Constant6/1 -> longitudinal control double PID/11(KD_PID_speed)
  speed_desire[m/s]/1 -> [speed_desire]
  control_predict_time[s]/1 -> [predict_time]
  host_speed[m/s]/1 -> [host_speed]
  host_vy[m/s]/1 -> [host_vy]
  host_y[m]/1 -> [host_y]
  [host_yaw_rate] -> lateral control LQR/6(host_yaw_dot[rad/s])
  yr_desire[m]/1 -> [yr_desire]
  kappar_desire[m^-1]/1 -> [kappar_desire]
  host_yawrate[rad/s]/1 -> [host_yaw_rate]
  [kappar_desire] -> lateral control LQR/10(kappar)
  [host_heading_xy] -> lateral control LQR/3(host_yaw[rad])
  [thetar_desire] -> lateral control LQR/9(thetar)
  lateral control LQR/4(LQR_ed) -> [LQR_ed]
  [speed_desire] -> longitudinal control double PID/2(speed_desire[m/s])
  host_vx[m/s]/1 -> [host_vx]
  [predict_time] -> lateral control LQR/11(predict_time)
  [host_speed] -> longitudinal control double PID/4(host_speed[m/s])
  Constant4/1 -> longitudinal control double PID/9(KP_PID_speed)
  Constant5/1 -> longitudinal control double PID/10(KI_PID_speed)
  Constant3/1 -> longitudinal control double PID/8(KD_PID_distance)
  Constant/1 -> longitudinal control double PID/6(KP_PID_distance)
  lateral control LQR/3(LQR_s_dot[m/s]) -> [LQR_s_dot]
  [LQR_ed] -> understeer compensate/2(lateral err)
  host_heading_xy[rad]/1 -> [host_heading_xy]
  lateral control LQR/2(LQR_es[m]) -> [LQR_es]
  [host_vy] -> lateral control LQR/5(host_vy[m/s])
  xr_desire[m]/1 -> [xr_desire]
  [LQR_angle] -> understeer compensate/1(LQR_angle)
  [yr_desire] -> lateral control LQR/8(yr)
  [LQR_s_dot] -> longitudinal control double PID/5(host_s_dot[m/s])
  [host_y] -> lateral control LQR/2(host_y[m])
  accelerate_desire[m/s^2]/1 -> [accelerate_desire]
  [xr_desire] -> lateral control LQR/7(xr)
  [host_x] -> lateral control LQR/1(host_x[m])
  [accelerate_desire] -> longitudinal control double PID/3(accelerate desire[m/s^2])
  Constant1/1 -> longitudinal control double PID/7(KI_PID_distance)
  thetar_desire[rad]/1 -> [thetar_desire]
  [host_vx] -> lateral control LQR/4(host_vx[m/s])
  lateral control LQR/1(LQR_angle[rad]) -> [LQR_angle]
  understeer compensate/1(LQR_final_angle) -> [LQR_final_angle]
  host_x[m]/1 -> [host_x]

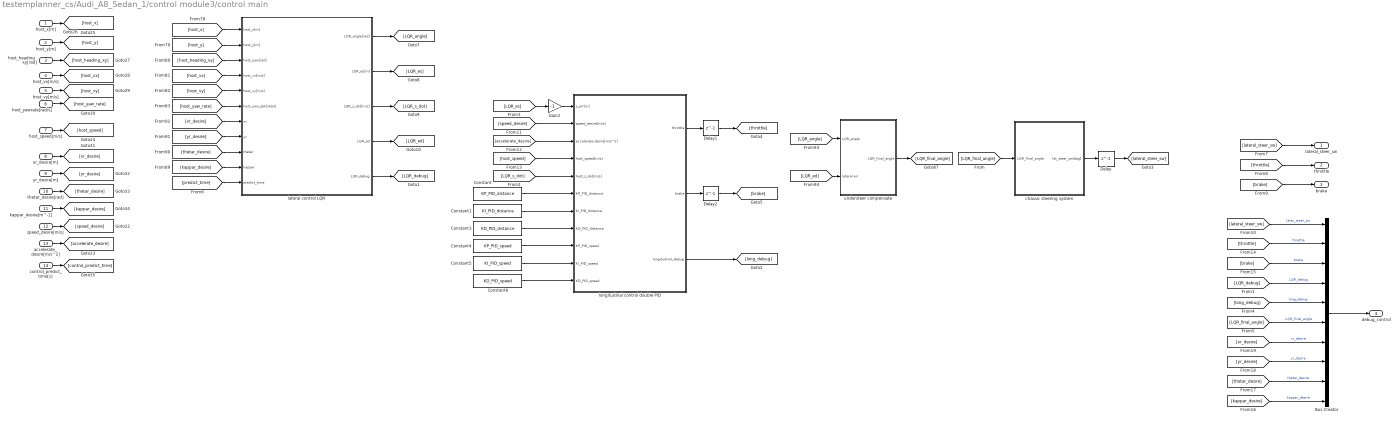
== system testemplanner_cs/Audi_A8_Sedan_1/control module3/control main ==
  host_x[m] : Inport
  host_y[m] : Inport  Port=2
  host_heading_xy[rad] : Inport  Port=3
  host_vx[m/s] : Inport  Port=4
  host_vy[m/s] : Inport  Port=5
  host_yawrate[rad/s] : Inport  Port=6
  host_speed[m/s] : Inport  Port=7
  xr_desire[m] : Inport  Port=8
  yr_desire[m] : Inport  Port=9
  thetar_desire[rad] : Inport  Port=10
  kappar_desire[m^-1] : Inport  Port=11
  speed_desire[m/s] : Inport  Port=12
  accelerate_desire[m/s^2] : Inport  Port=13
  control_predict_time[s] : Inport  Port=14
  Bus Creator : BusCreator  Inputs=10
  Constant : Constant  Value=KP_PID_distance
  Constant1 : Constant  Value=KI_PID_distance
  Constant3 : Constant  Value=KD_PID_distance
  Constant4 : Constant  Value=KP_PID_speed
  Constant5 : Constant  Value=KI_PID_speed
  Constant6 : Constant  Value=KD_PID_speed
  Delay : Delay  DelayLength=1
  Delay1 : Delay  DelayLength=1
  Delay2 : Delay  DelayLength=1
  Gain2 : Gain  Gain=-1
  chassic steering system : Subsystem
  lateral control LQR : Subsystem
  longitudinal control double PID : Subsystem
  understeer compensate : Subsystem
  lateral_steer_sw : Outport
  throttle : Outport  Port=2
  brake : Outport  Port=3
  debug_control : Outport  Port=4
  wires:
  [kappar_desire] -> Bus Creator/10  "kappar_desire"
  [thetar_desire] -> Bus Creator/9  "thetar_desire"
  [yr_desire] -> Bus Creator/8  "yr_desire"
  [xr_desire] -> Bus Creator/7  "xr_desire"
  Bus Creator/1 -> debug_control/1
  [LQR_final_angle] -> Bus Creator/6  "LQR_final_angle"
  [long_debug] -> Bus Creator/5  "long_debug"
  [LQR_debug] -> Bus Creator/4  "LQR_debug"
  [brake] -> Bus Creator/3  "brake"
  [throttle] -> Bus Creator/2  "throttle"
  [lateral_steer_sw] -> Bus Creator/1  "later_steer_sw"
  [brake] -> brake/1
  [throttle] -> throttle/1
  [lateral_steer_sw] -> lateral_steer_sw/1
  Delay2/1 -> [brake]
  Delay1/1 -> [throttle]
  Delay/1 -> [lateral_steer_sw]
  longitudinal control double PID/3(longitudinal_debug) -> [long_debug]
  lateral control LQR/5(LQR_debug) -> [LQR_debug]
  longitudinal control double PID/2(brake) -> Delay2/1
  longitudinal control double PID/1(throttle) -> Delay1/1
  chassic steering system/1(lat_steer_sw[deg]) -> Delay/1
  [LQR_final_angle] -> chassic steering system/1(LQR_final_angle)
  [LQR_es] -> Gain2/1
  Gain2/1 -> longitudinal control double PID/1(s_err[m])
  Constant6/1 -> longitudinal control double PID/11(KD_PID_speed)
  speed_desire[m/s]/1 -> [speed_desire]
  control_predict_time[s]/1 -> [control_predict_time]
  host_speed[m/s]/1 -> [host_speed]
  host_vy[m/s]/1 -> [host_vy]
  host_y[m]/1 -> [host_y]
  [host_yaw_rate] -> lateral control LQR/6(host_yaw_dot[rad/s])
  yr_desire[m]/1 -> [yr_desire]
  kappar_desire[m^-1]/1 -> [kappar_desire]
  host_yawrate[rad/s]/1 -> [host_yaw_rate]
  [kappar_desire] -> lateral control LQR/10(kappar)
  [host_heading_xy] -> lateral control LQR/3(host_yaw[rad])
  [thetar_desire] -> lateral control LQR/9(thetar)
  lateral control LQR/4(LQR_ed) -> [LQR_ed]
  [speed_desire] -> longitudinal control double PID/2(speed_desire[m/s])
  host_vx[m/s]/1 -> [host_vx]
  [predict_time] -> lateral control LQR/11(predict_time)
  [host_speed] -> longitudinal control double PID/4(host_speed[m/s])
  Constant4/1 -> longitudinal control double PID/9(KP_PID_speed)
  Constant5/1 -> longitudinal control double PID/10(KI_PID_speed)
  Constant3/1 -> longitudinal control double PID/8(KD_PID_distance)
  Constant/1 -> longitudinal control double PID/6(KP_PID_distance)
  lateral control LQR/3(LQR_s_dot[m/s]) -> [LQR_s_dot]
  [LQR_ed] -> understeer compensate/2(lateral err)
  host_heading_xy[rad]/1 -> [host_heading_xy]
  lateral control LQR/2(LQR_es[m]) -> [LQR_es]
  [host_vy] -> lateral control LQR/5(host_vy[m/s])
  xr_desire[m]/1 -> [xr_desire]
  [LQR_angle] -> understeer compensate/1(LQR_angle)
  [yr_desire] -> lateral control LQR/8(yr)
  [LQR_s_dot] -> longitudinal control double PID/5(host_s_dot[m/s])
  [host_y] -> lateral control LQR/2(host_y[m])
  accelerate_desire[m/s^2]/1 -> [accelerate_desire]
  [xr_desire] -> lateral control LQR/7(xr)
  [host_x] -> lateral control LQR/1(host_x[m])
  [accelerate_desire] -> longitudinal control double PID/3(accelerate desire[m/s^2])
  Constant1/1 -> longitudinal control double PID/7(KI_PID_distance)
  thetar_desire[rad]/1 -> [thetar_desire]
  [host_vx] -> lateral control LQR/4(host_vx[m/s])
  lateral control LQR/1(LQR_angle[rad]) -> [LQR_angle]
  understeer compensate/1(LQR_final_angle) -> [LQR_final_angle]
  host_x[m]/1 -> [host_x]
